simulink model "height_sim"  (R2023b)
settings: Solver=FixedStepAuto  StartTime=0.0  StopTime=37  FixedStep=0.1  RelTol=1e-3
values from neighbouring files (symbols this model uses):
  x_ref = x_ref.Data    [plot.m]
  y_ref = y_ref.Data    [plot.m]
  yaw_ref = yaw_ref.Data    [plot.m]
  z_ref = z_ref.Data    [plot.m]
undefined symbols (not defined in the file or in its folder): angdiff
settings Model: Creator=hampu  LastModifiedBy=hampu

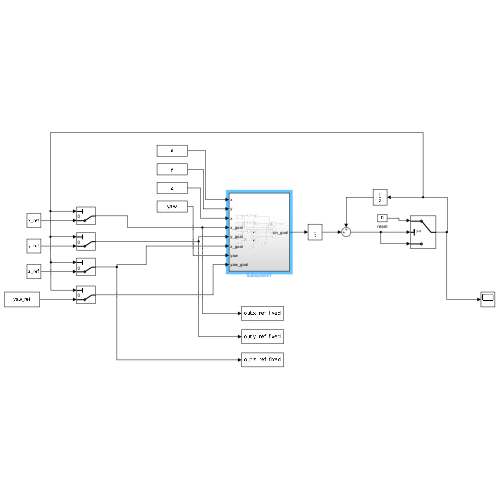
[thumbnail: Simulink's stored preview of the top-level diagram]
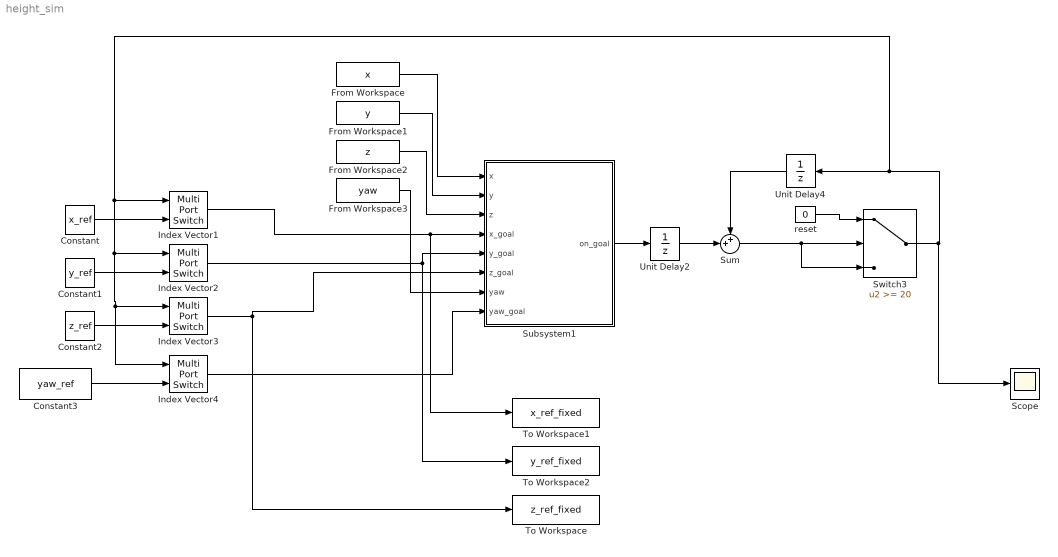
== system height_sim ==
  Constant : Constant  Value=x_ref
  Constant1 : Constant  Value=y_ref
  Constant2 : Constant  Value=z_ref
  Constant3 : Constant  Value=yaw_ref
  From Workspace : FromWorkspace  VariableName=x
  From Workspace1 : FromWorkspace  VariableName=y
  From Workspace2 : FromWorkspace  VariableName=z
  From Workspace3 : FromWorkspace  VariableName=yaw
  Index Vector{1..4} (4 alike) : MultiPortSwitch  DataPortOrder=Zero-based contiguous  Inputs=1  zeroidx=on  SaturateOnIntegerOverflow=off  InputSameDT=off
  Scope : Scope
  Subsystem1 : Subsystem
  Sum : Sum  Inputs=++|
  Switch3 : Switch  Threshold=20  SaturateOnIntegerOverflow=off  InputSameDT=off
  To Workspace : ToWorkspace  VariableName=z_ref_fixed  SaveFormat=Timeseries  SampleTime=-1
  To Workspace1 : ToWorkspace  VariableName=x_ref_fixed  SaveFormat=Timeseries  SampleTime=-1
  To Workspace2 : ToWorkspace  VariableName=y_ref_fixed  SaveFormat=Timeseries  SampleTime=-1
  Unit Delay2 : UnitDelay  SampleTime=-1  HasFrameUpgradeWarning=on
  Unit Delay4 : UnitDelay  SampleTime=-1  HasFrameUpgradeWarning=on
  reset : Constant  Value=0  VectorParams1D=off
  wires:
  Constant/1 -> Index Vector1/2
  From Workspace/1 -> Subsystem1/1(x)
  From Workspace1/1 -> Subsystem1/2(y)
  Sum/1 -> Switch3/2, Switch3/3
  From Workspace2/1 -> Subsystem1/3(z)
  Constant3/1 -> Index Vector4/2
  reset/1 -> Switch3/1
  Constant1/1 -> Index Vector2/2
  Constant2/1 -> Index Vector3/2
  From Workspace3/1 -> Subsystem1/7(yaw)
  Subsystem1/1(on_goal) -> Unit Delay2/1
  Unit Delay2/1 -> Sum/2
  Unit Delay4/1 -> Sum/1
  Switch3/1 -> Scope/1, Index Vector4/1, Index Vector3/1, Index Vector2/1, Index Vector1/1, Unit Delay4/1
  Index Vector1/1 -> To Workspace1/1, Subsystem1/4(x_goal)
  Index Vector2/1 -> Subsystem1/5(y_goal), To Workspace2/1
  Index Vector3/1 -> To Workspace/1, Subsystem1/6(z_goal)
  Index Vector4/1 -> Subsystem1/8(yaw_goal)

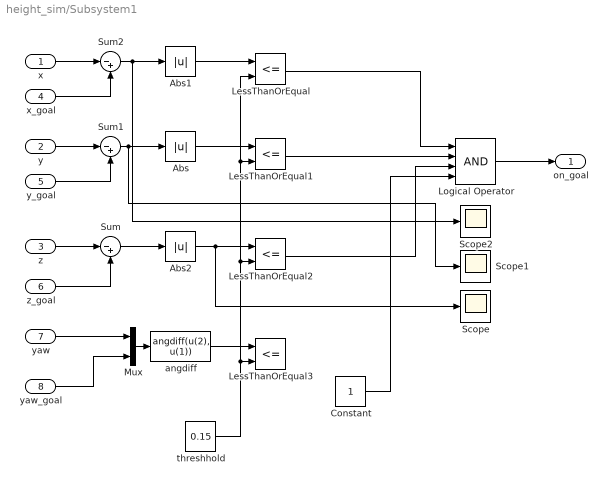
== system height_sim/Subsystem1 ==
  x : Inport
  y : Inport  Port=2
  z : Inport  Port=3
  x_goal : Inport  Port=4
  y_goal : Inport  Port=5
  z_goal : Inport  Port=6
  yaw : Inport  Port=7
  yaw_goal : Inport  Port=8  PortDimensions=1
  Abs : Abs  SaturateOnIntegerOverflow=off
  Abs1 : Abs  SaturateOnIntegerOverflow=off
  Abs2 : Abs  SaturateOnIntegerOverflow=off
  Constant : Constant
  LessThanOrEqual{,1..3} (4 alike) : RelationalOperator  Operator=<=  OutDataTypeStr=boolean  RndMeth=Simplest  InputSameDT=off
  Logical Operator : Logic  Inputs=4  AllPortsSameDT=off  OutDataTypeStr=boolean
  Mux : Mux  Inputs=2
  Scope : Scope
  Scope1 : Scope
  Scope2 : Scope
  Sum : Sum  Inputs=|-+
  Sum1 : Sum  Inputs=|-+
  Sum2 : Sum  Inputs=|-+
  angdiff : MATLABFcn  MATLABFcn=angdiff(u(2), u(1))
  threshhold : Constant  Value=0.15
  on_goal : Outport
  wires:
  z/1 -> Sum/1
  y/1 -> Sum1/1
  x/1 -> Sum2/1
  x_goal/1 -> Sum2/2
  y_goal/1 -> Sum1/2
  z_goal/1 -> Sum/2
  Sum2/1 -> Scope2/1, Abs1/1
  Sum1/1 -> Scope1/1, Abs/1
  Sum/1 -> Abs2/1
  Logical Operator/1 -> on_goal/1
  Abs1/1 -> LessThanOrEqual/1
  Abs/1 -> LessThanOrEqual1/1
  Abs2/1 -> Scope/1, LessThanOrEqual2/1
  threshhold/1 -> LessThanOrEqual3/2, LessThanOrEqual/2, LessThanOrEqual1/2, LessThanOrEqual2/2
  LessThanOrEqual/1 -> Logical Operator/1
  LessThanOrEqual1/1 -> Logical Operator/2
  LessThanOrEqual2/1 -> Logical Operator/3
  Mux/1 -> angdiff/1
  angdiff/1 -> LessThanOrEqual3/1
  Constant/1 -> Logical Operator/4
  yaw/1 -> Mux/1
  yaw_goal/1 -> Mux/2
